simulink model "MIL4L3_SW6_V1_20220211"  (R2018b)
settings: Solver=FixedStepAuto  StartTime=0.0  StopTime=inf  FixedStep=0.001  RelTol=1e-3
PreLoadFcn:
  | A0_MILtest;
undefined symbols (not defined in the file or in its folder): Clb_ICADirect_LaneDisp_StateFive, Clb_ICADirect_LaneDisp_StateFour, Clb_ICADirect_LaneDisp_StateOne, Clb_ICADirect_LaneDisp_StateThree, Clb_ICADirect_LaneDisp_StateTwo, Clb_ICADirect_LaneDisp_StateZero, Clb_ICADirect_LaneDispSW, Clb_ICADirect_TrnLghtsCom_Switch, Clb_ICADirect_TrnLghtsCom_Value, Clb_ICADirect_TrnLghtsCrtl_Inhb, IMAP_Clb_ACU_Driver_Belt, IMAP_Clb_ACU_Driver_Belt_Over, IMAP_Clb_ACU_Passenger_Belt, IMAP_Clb_ACU_Passenger_Belt_Over, IMAP_Clb_ACU_RearLeft_Belt, IMAP_Clb_ACU_RearLeft_Belt_Over, IMAP_Clb_ACU_RearMiddle_Belt, IMAP_Clb_ACU_RearMiddle_Belt_Over, IMAP_Clb_ACU_RearRight_Belt, IMAP_Clb_ACU_RearRight_Belt_Over, IMAP_Clb_AEB_Switch, IMAP_Clb_AEB_Switch_Over, IMAP_Clb_ALC_TLC_Mode, IMAP_Clb_ALC_TLC_Mode_Over, IMAP_Clb_BCM_Battery_Voltage, IMAP_Clb_BCM_Battery_Voltage_Over, IMAP_Clb_BCM_BrakeLamp_State, IMAP_Clb_BCM_BrakeLamp_State_Over, IMAP_Clb_BCM_CHMSL_Status, IMAP_Clb_BCM_CHMSL_Status_Over, IMAP_Clb_BCM_Door_Lock_State, IMAP_Clb_BCM_Door_Lock_State_Over, IMAP_Clb_BCM_FrontWiper_State, IMAP_Clb_BCM_FrontWiper_State_Over, IMAP_Clb_BCM_FrontWiper_Switch, IMAP_Clb_BCM_FrontWiper_Switch_Over, IMAP_Clb_BCM_HazardLamp, IMAP_Clb_BCM_HazardLamp_Over, IMAP_Clb_BCM_HazardLamp_Switch, IMAP_Clb_BCM_HazardLamp_Switch_Over, IMAP_Clb_BCM_HighBeam_State, IMAP_Clb_BCM_HighBeam_State_Over, IMAP_Clb_BCM_Ignition_State, IMAP_Clb_BCM_Ignition_State_Over, IMAP_Clb_BCM_IHBC_Enabled, IMAP_Clb_BCM_IHBC_Enabled_Over, IMAP_Clb_BCM_Left_Light, IMAP_Clb_BCM_Left_Light_Over, IMAP_Clb_BCM_LeftTurn_Switch, IMAP_Clb_BCM_LeftTurn_Switch_Over, IMAP_Clb_BCM_LF_Door_State, IMAP_Clb_BCM_LF_Door_State_Over, IMAP_Clb_BCM_LowBeam_State, IMAP_Clb_BCM_LowBeam_State_Over, IMAP_Clb_BCM_LR_Door_State, IMAP_Clb_BCM_LR_Door_State_Over, IMAP_Clb_BCM_RF_Door_State, IMAP_Clb_BCM_RF_Door_State_Over, IMAP_Clb_BCM_Right_Light, IMAP_Clb_BCM_Right_Light_Over ... (+547)
libraries: CarMaker4SL x2153, simulink x292, dspstat3 x3, canmsglib x2, simulink_extras x1
(part 48 of 52)

== system MIL4L3_SW6_V1_20220211/CarMaker/VehicleControl/Function/LKA/LKAS1/LL/LLOn/LL State Determination (LLStateDet)/LL State Machine Conditions (LLSMCon)/Enable Condition (EnaC)/LKA Own Condition (LKAOwnC)/Vehicle Position Check (VehPosChk)1 ==
  VehPosChk_LaneWidth : Inport
  VehPosChk_bsDvtInfo : Inport  Port=2
  VehPosChk_LKALineMax : Inport  Port=3
  VehPosChk_CarWidth : Inport  Port=4
  VehPosChk_lWarnLineMax_C : Inport  Port=5
  VehPosChk_lWarnLineMin_C : Inport  Port=6
  Bus Selector : BusSelector  OutputSignals=ILftDvt,IRgtDvt
  Logical Operator : Logic  AllPortsSameDT=off  OutDataTypeStr=boolean
  Logical Operator1 : Logic  Operator=OR  AllPortsSameDT=off  OutDataTypeStr=boolean
  Relational Operator1 : RelationalOperator  OutDataTypeStr=boolean  RndMeth=Nearest
  Relational Operator2 : RelationalOperator  OutDataTypeStr=boolean  RndMeth=Nearest
  Relational Operator3 : RelationalOperator  Operator=<=  OutDataTypeStr=boolean  RndMeth=Nearest
  Relational Operator4 : RelationalOperator  Operator=<=  OutDataTypeStr=boolean  RndMeth=Nearest
  Subsystem : Subsystem
  VehPosChk_stVehPosChk : Outport
  VehPosChk_stVehExLane : Outport  Port=2
  wires:
  Bus Selector/1 -> Relational Operator4/1, Relational Operator1/1  "<ILftDvt>"
  Bus Selector/2 -> Relational Operator2/1, Relational Operator3/1  "<IRgtDvt>"
  Relational Operator1/1 -> Logical Operator/1
  Relational Operator2/1 -> Logical Operator/2
  Logical Operator/1 -> VehPosChk_stVehPosChk/1
  VehPosChk_bsDvtInfo/1 -> Bus Selector/1
  Subsystem/1(EnableLine) -> Relational Operator1/2, Relational Operator2/2
  VehPosChk_lWarnLineMax_C/1 -> Subsystem/1(WarnLine_C)
  VehPosChk_LaneWidth/1 -> Subsystem/2(LaneWidth)
  Logical Operator1/1 -> VehPosChk_stVehExLane/1
  Relational Operator3/1 -> Logical Operator1/2
  VehPosChk_lWarnLineMin_C/1 -> Relational Operator3/2, Relational Operator4/2
  Relational Operator4/1 -> Logical Operator1/1
  VehPosChk_LKALineMax/1 -> Subsystem/3(VehPosChk_LKALineMax)
  VehPosChk_CarWidth/1 -> Subsystem/4(VehPosChk_CarWidth)

== system MIL4L3_SW6_V1_20220211/CarMaker/VehicleControl/Function/LKA/LKAS1/LL/LLOn/LL State Determination (LLStateDet)/LL State Machine Conditions (LLSMCon)/Enable Condition (EnaC)/Lane Condition (LaneC)/Lane C1 Detection (LaneC1Det) ==
  LaneWDet_facmL0C1 : Inport
  LaneWDet_facmR0C1 : Inport  Port=2
  Abs : Abs
  Add : Sum  Inputs=+-  OutDataTypeStr=single
  Compare To Constant1 : simulink/Logic and Bit Operations/Compare To Constant  relop=<=  const=0.025  OutDataTypeStr=boolean
  LaneC1Det_stLaneC1DetFlg : Outport
  wires:
  LaneWDet_facmR0C1/1 -> Add/2
  LaneWDet_facmL0C1/1 -> Add/1
  Add/1 -> Abs/1
  Compare To Constant1/1 -> LaneC1Det_stLaneC1DetFlg/1
  Abs/1 -> Compare To Constant1/1

== system MIL4L3_SW6_V1_20220211/CarMaker/VehicleControl/Function/LKA/LKAS1/LL/LLOn/LL State Determination (LLStateDet)/LL State Machine Conditions (LLSMCon)/Enable Condition (EnaC)/Lane Condition (LaneC)/Lane Condition Synthesis (LaneCSyn) ==
  LaneCSyn_stLaneQlECFlg : Inport
  LaneCSyn_stLaneWDetFlg : Inport  Port=2
  LaneCSyn_stLaneCrvtDetFlg : Inport  Port=3
  LaneCSyn_stLaneC1DetFlg : Inport  Port=4
  Logical Operator3 : Logic  Inputs=4  AllPortsSameDT=off  OutDataTypeStr=boolean
  LaneCSyn_stLaneCSyn : Outport
  wires:
  LaneCSyn_stLaneQlECFlg/1 -> Logical Operator3/1
  LaneCSyn_stLaneCrvtDetFlg/1 -> Logical Operator3/3
  Logical Operator3/1 -> LaneCSyn_stLaneCSyn/1
  LaneCSyn_stLaneWDetFlg/1 -> Logical Operator3/2
  LaneCSyn_stLaneC1DetFlg/1 -> Logical Operator3/4

== system MIL4L3_SW6_V1_20220211/CarMaker/VehicleControl/Function/LKA/LKAS1/LL/LLOn/LL State Determination (LLStateDet)/LL State Machine Conditions (LLSMCon)/Enable Condition (EnaC)/Lane Condition (LaneC)/Lane Curvature Detection (LaneCrvtDet) ==
  LaneCrvtDet_crPrvwCrvt : Inport
  LaneCrvtDet_crLaneCrvtMax_C : Inport  Port=2
  Abs : Abs
  Constant : Constant  Value=0  OutDataTypeStr=single  SampleTime=-1
  Interval Test Dynamic : simulink/Logic and Bit Operations/Interval Test Dynamic  IntervalClosedRight=on  IntervalClosedLeft=on  OutDataTypeStr=boolean
      settings: SourceProductName=Simulink  SourceProductBaseCode=SL
  LaneCrvtDet_stLaneCrvtDetFlg : Outport
  wires:
  Interval Test Dynamic/1 -> LaneCrvtDet_stLaneCrvtDetFlg/1
  LaneCrvtDet_crLaneCrvtMax_C/1 -> Interval Test Dynamic/1
  Constant/1 -> Interval Test Dynamic/3
  LaneCrvtDet_crPrvwCrvt/1 -> Abs/1
  Abs/1 -> Interval Test Dynamic/2

== system MIL4L3_SW6_V1_20220211/CarMaker/VehicleControl/Function/LKA/LKAS1/LL/LLOn/LL State Determination (LLStateDet)/LL State Machine Conditions (LLSMCon)/Enable Condition (EnaC)/Lane Condition (LaneC)/Lane Quality Enable Condition (LaneQlEC) ==
  LaneQlEC_stFacmL0Ql : Inport
  LaneQlEC_stFacmR0Ql : Inport  Port=2
  Compare To Constant : simulink/Logic and Bit Operations/Compare To Constant  relop=>  const=2  OutDataTypeStr=boolean
  Compare To Constant1 : simulink/Logic and Bit Operations/Compare To Constant  relop=>  const=2  OutDataTypeStr=boolean
  Logical Operator : Logic  AllPortsSameDT=off  OutDataTypeStr=boolean
  LaneQlEC_stLaneQlECFlg : Outport
  wires:
  LaneQlEC_stFacmL0Ql/1 -> Compare To Constant/1
  LaneQlEC_stFacmR0Ql/1 -> Compare To Constant1/1
  Compare To Constant/1 -> Logical Operator/1
  Compare To Constant1/1 -> Logical Operator/2
  Logical Operator/1 -> LaneQlEC_stLaneQlECFlg/1

== system MIL4L3_SW6_V1_20220211/CarMaker/VehicleControl/Function/LKA/LKAS1/LL/LLOn/LL State Determination (LLStateDet)/LL State Machine Conditions (LLSMCon)/Enable Condition (EnaC)/Lane Condition (LaneC)/Lane Width Detection (LaneWDet) ==
  LaneWDet_LaneWidth : Inport
  LaneWDet_lLaneWMax : Inport  Port=2
  LaneWDet_lLaneWMin : Inport  Port=3
  Abs1 : Abs
  Interval Test Dynamic : simulink/Logic and Bit Operations/Interval Test Dynamic  IntervalClosedRight=on  IntervalClosedLeft=on  OutDataTypeStr=boolean
      settings: SourceProductName=Simulink  SourceProductBaseCode=SL
  LaneWDet_stLaneWDetFlg : Outport
  wires:
  Interval Test Dynamic/1 -> LaneWDet_stLaneWDetFlg/1
  LaneWDet_lLaneWMax/1 -> Interval Test Dynamic/1
  LaneWDet_lLaneWMin/1 -> Interval Test Dynamic/3
  Abs1/1 -> Interval Test Dynamic/2
  LaneWDet_LaneWidth/1 -> Abs1/1

== system MIL4L3_SW6_V1_20220211/CarMaker/VehicleControl/Function/LKA/LKAS1/LL/LLOn/LL State Determination (LLStateDet)/LL State Machine Conditions (LLSMCon)/Enable Condition (EnaC)/Vehicle State Condition (VehStateC)/Emergency Light Enable Condition (EmgcyLghtEC) ==
  EmgcyLghtEC_bsStLampState : Inport
  Add : Sum
  Bus Selector : BusSelector  OutputSignals=BCM_Double_Light,BCM_Left_Light,BCM_Right_Light
  Compare To Constant : simulink/Logic and Bit Operations/Compare To Constant  relop=<=  const=0  OutDataTypeStr=boolean
  Compare To Constant1 : simulink/Logic and Bit Operations/Compare To Constant  relop=>=  const=3  OutDataTypeStr=boolean
  Compare To Constant2 : simulink/Logic and Bit Operations/Compare To Constant  relop=>  const=0  OutDataTypeStr=boolean
  Compare To Constant3 : simulink/Logic and Bit Operations/Compare To Constant  relop=>  const=0  OutDataTypeStr=boolean
  Constant : Constant  Value=3  OutDataTypeStr=single
  Constant1 : Constant  Value=-1  OutDataTypeStr=single
  Logical Operator : Logic  Operator=OR  Inputs=3  AllPortsSameDT=off  OutDataTypeStr=boolean
  Memory : Memory  InheritSampleTime=on
  Saturation : Saturate  UpperLimit=200  LowerLimit=-1
      settings: AttributesFormatString="Min = %<LowerLimit>  Max = %<UpperLimit>"
  Switch : Switch  Criteria=u2 > Threshold
  EmgcyLghtEC_stEmgcyLghtECFlg : Outport
  wires:
  Compare To Constant2/1 -> Logical Operator/2
  Compare To Constant1/1 -> Logical Operator/1
  EmgcyLghtEC_bsStLampState/1 -> Bus Selector/1
  Bus Selector/1 -> Compare To Constant1/1  "<BCM_Double_Light>"
  Bus Selector/2 -> Compare To Constant2/1  "<BCM_Left_Light>"
  Logical Operator/1 -> Switch/2
  Constant/1 -> Switch/1
  Constant1/1 -> Switch/3
  Switch/1 -> Add/1
  Add/1 -> Saturation/1
  Saturation/1 -> Compare To Constant/1, Memory/1
  Memory/1 -> Add/2
  Compare To Constant/1 -> EmgcyLghtEC_stEmgcyLghtECFlg/1
  Bus Selector/3 -> Compare To Constant3/1  "<BCM_Right_Light>"
  Compare To Constant3/1 -> Logical Operator/3

== system MIL4L3_SW6_V1_20220211/CarMaker/VehicleControl/Function/LKA/LKAS1/LL/LLOn/LL State Determination (LLStateDet)/LL State Machine Conditions (LLSMCon)/Enable Condition (EnaC)/Vehicle State Condition (VehStateC)/Gear Enable Condition (GearEC) ==
  GearEC_bsTCUState : Inport
  Bus Selector : BusSelector  OutputSignals=TCU_ActualGear
  Compare To Constant : simulink/Logic and Bit Operations/Compare To Constant  relop===  const=3  OutDataTypeStr=boolean
  GearEC_stGearECFlg : Outport
  wires:
  GearEC_bsTCUState/1 -> Bus Selector/1
  Bus Selector/1 -> Compare To Constant/1  "<TCU_ActualGear>"
  Compare To Constant/1 -> GearEC_stGearECFlg/1

== system MIL4L3_SW6_V1_20220211/CarMaker/VehicleControl/Function/LKA/LKAS1/LL/LLOn/LL State Determination (LLStateDet)/LL State Machine Conditions (LLSMCon)/Enable Condition (EnaC)/Vehicle State Condition (VehStateC)/Vehicle Speed Enable Condition (VehSpdEC) ==
  VehSpdEC_stDACMode : Inport
  VehSpdEC_vVehSpd : Inport  Port=2
  VehSpdEC_vLDWVehSpdMax_C : Inport  Port=3
  VehSpdEC_vLKAVehSpdMax_C : Inport  Port=4
  VehSpdEC_vVehSpdMin_C : Inport  Port=5
  Interval Test Dynamic : simulink/Logic and Bit Operations/Interval Test Dynamic  IntervalClosedRight=on  IntervalClosedLeft=on  OutDataTypeStr=boolean
      settings: SourceProductName=Simulink  SourceProductBaseCode=SL
  Switch : Switch  Threshold=2
  VehSpdEC_stVehSpdECFlg : Outport
  wires:
  VehSpdEC_vVehSpd/1 -> Interval Test Dynamic/2
  VehSpdEC_vVehSpdMin_C/1 -> Interval Test Dynamic/3
  Interval Test Dynamic/1 -> VehSpdEC_stVehSpdECFlg/1
  VehSpdEC_stDACMode/1 -> Switch/2
  VehSpdEC_vLKAVehSpdMax_C/1 -> Switch/1
  Switch/1 -> Interval Test Dynamic/1
  VehSpdEC_vLDWVehSpdMax_C/1 -> Switch/3

== system MIL4L3_SW6_V1_20220211/CarMaker/VehicleControl/Function/LKA/LKAS1/LL/LLOn/LL State Determination (LLStateDet)/LL State Machine Conditions (LLSMCon)/Enable Condition (EnaC)/Vehicle State Condition (VehStateC)/Vehicle State Condition Synthesis (VehStateCSyn) ==
  VehStateCSyn_stVehSpdECFlg : Inport
  VehStateCSyn_stEmgcyLghtECFlg : Inport  Port=2
  VehStateCSyn_stGearECFlg : Inport  Port=3
  Logical Operator : Logic  Inputs=3  AllPortsSameDT=off  OutDataTypeStr=boolean
  VehStateCSyn_stVehStateCSyn : Outport
  wires:
  VehStateCSyn_stVehSpdECFlg/1 -> Logical Operator/1
  VehStateCSyn_stGearECFlg/1 -> Logical Operator/3
  Logical Operator/1 -> VehStateCSyn_stVehStateCSyn/1
  VehStateCSyn_stEmgcyLghtECFlg/1 -> Logical Operator/2

== system MIL4L3_SW6_V1_20220211/CarMaker/VehicleControl/OMAP/OMAP1/Runnable_OMAP_10ms_sys/OMAP_Module/ICA_Direct_G59/ICA_Define/Subsystem1/Dspl/DsplPrcs/Icon ==
  note: 0：灭
      | 1：灰
      | 2：绿
      | 3：橙
      | 4：红
  note: 显示0条件：多车道模式选择ICA；
      | 显示1条件（灰色）：多车道模式选择TCL或ALC，THState~=0；
      | 显示2条件（绿色，不带AUTO）：多车道模式选择TLC，速度大于变道允许门槛值，THState=3；
      | 显示3条件（绿色，带AUTO）：多车道模式选择ALC，速度大于变道允许门槛值，THState=3；
      | 显示4条件（橙色）：多车道模式选择TLC或者ALC，速度大于变道允许门槛值，THState=4
      | 显示5条件（红色）：多车道模式选择TLC或者ALC，速度大于变道允许门槛值，THState=5
      | 之所以把速度条件加进来，其实是考虑到多车道功能的激活隐含了速度要大于某一门槛值这个条件
  note: 0：Default Value
      | 1：HWA Unavailable（未启用）
      | 2：HWA_TLC（触发式变道）
      | 3：HWA_ALC（主动变道）
      | 4：HWA_SL_SRR_Fail（硬件故障-功能无法开启或降级）
      | 5：HWA_Error（系统故障）
      | 6：Reserved（保留）
  note: 0 ：可以从降级回到正常，
      | 1 ：不可以从降级回到正常
  note: ACC_State【0：初始化；1：关闭；2：禁止；3：等待；4：激活；5：Override；6：只能制动；7：Cancel键退出；8：OFF键退出；15：故障】
  Icon_stTHState : Inport
  Icon_stACCState : Inport  Port=2
  Icon_dDgrdIconWarnHiDurnum : Inport  Port=3
  Icon_dDgrdIconWarnLoDurnum : Inport  Port=4
  Icon_dDgrdIconWarnflag : Inport  Port=5
  Icon_stTLC_ALCmodeSW : Inport  Port=6
  Icon_stLC_SpdCndtFlg : Inport  Port=7
  Bus Creator : BusCreator  Inputs=2
  Constant : Constant  Value=OMAP_ICA_iconSTATE0  OutDataTypeStr=uint16
  Constant1 : Constant  Value=OMAP_ICA_iconSTATE1  OutDataTypeStr=uint16
  Constant10 : Constant  Value=5  OutDataTypeStr=uint16
  Constant11 : Constant  OutDataTypeStr=uint16
  Constant12 : Constant  Value=0  OutDataTypeStr=uint16
  Constant13 : Constant  Value=OMAP_ICA_iconSTATE6  OutDataTypeStr=uint16
  Constant14 : Constant  Value=OMAP_ICA_iconSTATE7  OutDataTypeStr=uint16
  Constant15 : Constant  Value=OMAP_ICA_iconSTATE8  OutDataTypeStr=uint16
  Constant16 : Constant  Value=OMAP_ICA_iconSTATE4  OutDataTypeStr=uint16
  Constant2 : Constant  Value=OMAP_ICA_iconSTATE2  OutDataTypeStr=uint16
  Constant3 : Constant  Value=OMAP_ICA_iconSTATE3  OutDataTypeStr=uint16
  Constant4 : Constant  Value=OMAP_ICA_iconSTATE4  OutDataTypeStr=uint16
  Constant5 : Constant  Value=OMAP_ICA_iconSTATE5  OutDataTypeStr=uint16
  Constant6 : Constant  OutDataTypeStr=boolean
  Constant7 : Constant  Value=2  OutDataTypeStr=uint16
  Constant8 : Constant  Value=3  OutDataTypeStr=uint16
  Constant9 : Constant  Value=4  OutDataTypeStr=uint16
  If : If  NumInputs=2  IfExpression=u1==0  ElseIfExpressions=u1==1,u1==2,u1==3,u1==4,u1==5,u1==6,u1==7,(u1==8)&(u2~=4&u2~=5&u2~=6),(u1==8)&(u2==4|u2==5|u2==6)
  If Action Subsystem : Subsystem  TreatAsAtomicUnit=on
  If Action Subsystem1 : Subsystem  TreatAsAtomicUnit=on
  If Action Subsystem10 : Subsystem  TreatAsAtomicUnit=on
  If Action Subsystem11 : Subsystem  TreatAsAtomicUnit=on
  If Action Subsystem12 : Subsystem  TreatAsAtomicUnit=on
  If Action Subsystem13 : Subsystem  TreatAsAtomicUnit=on
  If Action Subsystem14 : Subsystem  TreatAsAtomicUnit=on
  If Action Subsystem15 : Subsystem  TreatAsAtomicUnit=on
  If Action Subsystem16 : Subsystem  TreatAsAtomicUnit=on
  If Action Subsystem2 : Subsystem  TreatAsAtomicUnit=on
  If Action Subsystem3 : Subsystem  TreatAsAtomicUnit=on
  If Action Subsystem4 : Subsystem  TreatAsAtomicUnit=on
  If Action Subsystem5 : Subsystem  TreatAsAtomicUnit=on
  If Action Subsystem6 : Subsystem  TreatAsAtomicUnit=on
  If Action Subsystem7 : Subsystem  TreatAsAtomicUnit=on
  If Action Subsystem8 : Subsystem  TreatAsAtomicUnit=on
  If Action Subsystem9 : Subsystem  TreatAsAtomicUnit=on
  If1 : If  IfExpression=u1 == 0
  If2 : If  NumInputs=3  IfExpression=u1==3&u2==2&u3==1  ElseIfExpressions=u1==3&u2==3&u3==1,u1==4&(u2==2|u2==3)&u3==1,u1==5&(u2==2|u2==3)&u3==1,u1~=0&(u2==2|u2==3)
  Merge : Merge  Inputs=11
  Merge1 : Merge
  Merge2 : Merge  Inputs=6
  Terminator : Terminator
  Terminator1 : Terminator
  Terminator2 : Terminator
  Unit Delay1 : UnitDelay  SampleTime=-1
  else : Subsystem  TreatAsAtomicUnit=on
  if : Subsystem  TreatAsAtomicUnit=on
  Icon_stIconDspl : Outport
  wires:
  Icon_stTHState/1 -> If2/1, If/1
  Icon_stACCState/1 -> If/2
  If/4 -> If Action Subsystem9/Action
  If/2 -> If Action Subsystem7/Action
  If/1 -> If Action Subsystem6/Action
  If/11 -> If Action Subsystem15/Action
  If/3 -> If Action Subsystem8/Action
  If/5 -> If Action Subsystem10/Action
  If Action Subsystem9/1(Out1) -> Merge/4
  Merge/1 -> Bus Creator/1, Unit Delay1/1  "Icon_stICAIcon"
  Unit Delay1/1 -> If Action Subsystem12/1(In1), If Action Subsystem15/1(In1), If Action Subsystem13/1(In1)
  If Action Subsystem6/1(Out1) -> Merge/1
  If Action Subsystem7/1(Out1) -> Merge/2
  If Action Subsystem8/1(Out1) -> Merge/3
  If Action Subsystem10/1(Out1) -> Merge/5
  If Action Subsystem11/1(Out1) -> Merge/6
  Constant/1 -> If Action Subsystem6/1(In1)
  Constant4/1 -> If Action Subsystem10/1(In1)
  Constant1/1 -> If Action Subsystem7/1(In1)
  Constant2/1 -> If Action Subsystem8/1(In1)
  If1/1 -> if/Action
  If1/2 -> else/Action
  Constant6/1 -> if/1(In1)
  if/1(Out1) -> Merge1/1
  Merge1/1 -> Terminator/1  "orange_enable"
  else/2(counter_status) -> Merge1/2
  Icon_dDgrdIconWarnflag/1 -> If1/1  "DgrdIconWarnflag"
  Icon_dDgrdIconWarnHiDurnum/1 -> else/1(HiDurnum)  "DgrdIconWarnHinum"
  Icon_dDgrdIconWarnLoDurnum/1 -> else/2(LoDurnum)  "DgrdIconWarnLonum"
  Icon_stTLC_ALCmodeSW/1 -> If2/2  "DgrdIconWarnLonum"
  Icon_stLC_SpdCndtFlg/1 -> If2/3  "DgrdIconWarnLonum"
  If2/1 -> If Action Subsystem/Action
  Constant7/1 -> If Action Subsystem/1(In1)
  If Action Subsystem/1(Out1) -> Merge2/1
  Constant8/1 -> If Action Subsystem1/1(In1)
  If2/2 -> If Action Subsystem1/Action
  If Action Subsystem1/1(Out1) -> Merge2/2
  Constant9/1 -> If Action Subsystem2/1(In1)
  If2/3 -> If Action Subsystem2/Action
  If Action Subsystem2/1(Out1) -> Merge2/3
  Constant10/1 -> If Action Subsystem3/1(In1)
  If2/4 -> If Action Subsystem3/Action
  If Action Subsystem3/1(Out1) -> Merge2/4
  Constant11/1 -> If Action Subsystem4/1(In1)
  If2/5 -> If Action Subsystem4/Action
  If Action Subsystem4/1(Out1) -> Merge2/5
  Constant12/1 -> If Action Subsystem5/1(In1)
  If2/6 -> If Action Subsystem5/Action
  If Action Subsystem5/1(Out1) -> Merge2/6
  Merge2/1 -> Bus Creator/2  "Icon_stHWAmode"
  Bus Creator/1 -> Icon_stIconDspl/1
  Constant3/1 -> If Action Subsystem9/1(In1)
  Constant5/1 -> If Action Subsystem11/1(In1)
  If/6 -> If Action Subsystem11/Action
  If/7 -> If Action Subsystem12/Action
  If Action Subsystem12/1(Out1) -> Merge/7
  If/8 -> If Action Subsystem13/Action
  If Action Subsystem13/1(Out1) -> Merge/8
  Constant15/1 -> If Action Subsystem14/1(In1)
  If/9 -> If Action Subsystem14/Action
  If Action Subsystem14/1(Out1) -> Merge/9
  If Action Subsystem15/1(Out1) -> Merge/11
  Constant13/1 -> Terminator1/1
  Constant14/1 -> Terminator2/1
  Constant16/1 -> If Action Subsystem16/1(In1)
  If/10 -> If Action Subsystem16/Action
  If Action Subsystem16/1(Out1) -> Merge/10

== system MIL4L3_SW6_V1_20220211/CarMaker/VehicleControl/OMAP/OMAP1/Runnable_OMAP_10ms_sys/OMAP_Module/ICA_Direct_G59/ICA_Define/Subsystem1/Dspl/DsplPrcs/Lane ==
  note: 变道但条件不满足的车道线显示：
      | 1、多车道模式为TLC或者ALC；
      | 1、转向灯已经打了；
      | 2、由于条件不满足，THmode无法跳到状态4（=1或2）；
      | 3、驾驶员没有自己打方向变道（通过接管信号判断），此条其实可以由THState=3覆盖
      | 4、THState在状态3
  note: ->1
  note: ->14
  note: ->2
  note: ->0
  note: 0是运动，1是静止
  Lane_stTHState : Inport
  Lane_stVehSty : Inport  Port=2
  Lane_facmL0Ql : Inport  Port=3
  Lane_facmR0Ql : Inport  Port=4
  Lane_facmL0Type : Inport  Port=5
  Lane_facmR0Type : Inport  Port=6
  Lane_stturn_lightState : Inport  Port=7
  Lane_stTLC_ALCmodeSW : Inport  Port=8
  Lane_stTkOvStChk : Inport  Port=9
  Bus Creator : BusCreator  Inputs=3
  Compare To Constant : simulink/Logic and Bit Operations/Compare To Constant  relop===  const=2  OutDataTypeStr=boolean
  Compare To Constant1 : simulink/Logic and Bit Operations/Compare To Constant  relop===  const=3  OutDataTypeStr=boolean
  Compare To Constant2 : simulink/Logic and Bit Operations/Compare To Constant  relop===  const=3  OutDataTypeStr=boolean
  Compare To Constant3 : simulink/Logic and Bit Operations/Compare To Constant  relop===  const=uint16(3)  OutDataTypeStr=boolean
  Compare To Constant4 : simulink/Logic and Bit Operations/Compare To Constant  relop===  const=uint16(3)  OutDataTypeStr=boolean
  Compare To Constant5 : simulink/Logic and Bit Operations/Compare To Constant  relop===  const=0  OutDataTypeStr=boolean
  Compare To Constant6 : simulink/Logic and Bit Operations/Compare To Constant  relop=~=  const=0  OutDataTypeStr=boolean
  Compare To Zero : simulink/Logic and Bit Operations/Compare To Zero  relop===  OutDataTypeStr=boolean
  Constant{,1,5,13} (4 alike) : Constant  Value=Clb_ICADirect_LaneDisp_StateZero  OutDataTypeStr=uint16
  Constant10 : Constant  OutDataTypeStr=uint16
  Constant11 : Constant  Value=16  OutDataTypeStr=uint16
  Constant12 : Constant  Value=0  OutDataTypeStr=uint16
  Constant14 : Constant  Value=Clb_ICADirect_LaneDisp_StateTwo  OutDataTypeStr=uint16
  Constant15 : Constant  Value=Clb_ICADirect_LaneDisp_StateFive  OutDataTypeStr=uint16
  Constant16 : Constant  Value=Clb_ICADirect_LaneDisp_StateThree  OutDataTypeStr=uint16
  Constant17 : Constant  Value=Clb_ICADirect_LaneDisp_StateFour  OutDataTypeStr=uint16
  Constant18 : Constant  Value=Clb_ICADirect_LaneDispSW  OutDataTypeStr=boolean
  Constant2 : Constant  Value=Clb_ICADirect_LaneDisp_StateTwo  OutDataTypeStr=uint16
  Constant3 : Constant  Value=15  OutDataTypeStr=uint16
  Constant4 : Constant  Value=Clb_ICADirect_LaneDisp_StateOne  OutDataTypeStr=uint16
  Constant6 : Constant  Value=Clb_ICADirect_LaneDisp_StateOne  OutDataTypeStr=uint16
  Constant7 : Constant  Value=3  OutDataTypeStr=uint16
  Constant8 : Constant  OutDataTypeStr=uint16
  Constant9 : Constant  Value=3  OutDataTypeStr=uint16
  Data Type Conversion{,1..7} (8 alike) : DataTypeConversion  OutDataTypeStr=uint16
  If : If  IfExpression=u1==0|u1==5  ElseIfExpressions=u1==3,(u1==1|u1==2|u1==4|u1==6|u1==7|u1==8)
  If1 : If  NumInputs=3  IfExpression=u1==0|u1==5  ElseIfExpressions=u1==3,u1==1|u1==4|(u2<3&u3<3),u2==3&u3==3,u2==3&u3<3,u2<3&u3==3
  Index Vector : MultiPortSwitch  DataPortOrder=Zero-based contiguous  Inputs=2  zeroidx=on
  Logical Operator : Logic  Operator=OR  AllPortsSameDT=off  OutDataTypeStr=boolean
  Logical Operator1 : Logic  Inputs=4  AllPortsSameDT=off  OutDataTypeStr=boolean
  Merge : Merge  Inputs=4
  Merge1 : Merge  Inputs=4
  Merge2 : Merge  Inputs=4
  Merge3 : Merge  Inputs=7
  Multiport Switch : MultiPortSwitch  Inputs=2  DataPortIndices={1,2}  DataPortForDefault=Additional data port  DiagnosticForDefault=None
  Subsystem : Subsystem
  Switch : Switch  Criteria=u2 ~= 0
  Switch1 : Switch  Criteria=u2 ~= 0
  Switch2 : Switch  Criteria=u2 ~= 0
  Switch3 : Switch  Criteria=u2 > Threshold  OutDataTypeStr=uint16
  both_blue : Subsystem  TreatAsAtomicUnit=on
  both_gray1 : Subsystem  TreatAsAtomicUnit=on
  not_dispay : Subsystem  TreatAsAtomicUnit=on
  not_dispay1 : Subsystem  TreatAsAtomicUnit=on
  not_dispay2 : Subsystem  TreatAsAtomicUnit=on
  not_dispay3 : Subsystem  TreatAsAtomicUnit=on
  not_dispay4 : Subsystem  TreatAsAtomicUnit=on
  not_dispay5 : Subsystem  TreatAsAtomicUnit=on
  not_dispay6 : Subsystem  TreatAsAtomicUnit=on
  not_dispay7 : Subsystem  TreatAsAtomicUnit=on
  not_display2 : Subsystem  TreatAsAtomicUnit=on
  Lane_stLaneDspl : Outport
  wires:
  If/1 -> not_dispay/Action
  Lane_stVehSty/1 -> Data Type Conversion1/1
  both_gray1/1(Out1) -> Merge/3
  Lane_facmR0Type/1 -> Compare To Constant4/1
  Lane_facmR0Ql/1 -> If1/3
  Switch/1 -> Lane_stLaneDspl/1
  Compare To Zero/1 -> Switch/2, Subsystem/Enable
  Compare To Constant3/1 -> Switch1/2
  not_display2/1(Out1) -> Merge/4
  Lane_facmL0Type/1 -> Compare To Constant3/1
  Lane_facmL0Ql/1 -> If1/2
  Data Type Conversion5/1 -> Bus Creator/3  "stR0DispType"
  not_dispay/1(Out1) -> Merge/1
  [stL0DispType] -> both_blue/2(In2)
  Compare To Constant4/1 -> Switch2/2
  Constant2/1 -> both_blue/1(In1)
  both_blue/1(Out1) -> Merge/2
  Switch1/1 -> [stL0DispType]
  Subsystem/1(Out1) -> Switch/3
  [stR0DispType] -> both_blue/3(In3)
  Data Type Conversion4/1 -> Bus Creator/2  "stL0DispType"
  Constant8/1 -> Switch1/3
  Merge2/1 -> Data Type Conversion5/1
  Switch2/1 -> [stR0DispType]
  both_blue/3(Out3) -> Merge2/2
  Lane_stTHState/1 -> Data Type Conversion3/1
  Constant9/1 -> Switch2/1
  Merge1/1 -> Data Type Conversion4/1
  not_display2/3(Out3) -> Merge2/4
  Constant10/1 -> Switch2/3
  If/3 -> both_gray1/Action
  not_dispay/3(Out3) -> Merge2/1
  Constant7/1 -> Switch1/1
  If/2 -> both_blue/Action
  [stL0DispType] -> both_gray1/2(In2)
  If/4 -> not_display2/Action
  not_display2/2(Out2) -> Merge1/4
  Constant/1 -> not_dispay/1(In1)
  Bus Creator/1 -> Switch/1, Subsystem/1(In1)
  both_gray1/2(Out2) -> Merge1/3
  [stR0DispType] -> both_gray1/3(In3)
  Merge/1 -> Index Vector/2  "stLaneDspl"
  Data Type Conversion1/1 -> Compare To Zero/1
  [stR0DispType] -> not_dispay/3(In3)
  not_dispay/2(Out2) -> Merge1/1
  [stL0DispType] -> not_dispay/2(In2)
  [stL0DispType] -> not_display2/2(In2)
  Constant5/1 -> not_display2/1(In1)
  Constant4/1 -> both_gray1/1(In1)
  both_gray1/3(Out3) -> Merge2/3
  both_blue/2(Out2) -> Merge1/2
  [stR0DispType] -> not_display2/3(In3)
  Data Type Conversion/1 -> Bus Creator/1  "stLaneDspl"
  Switch3/1 -> Data Type Conversion/1
  Data Type Conversion2/1 -> Compare To Constant1/1, Compare To Constant/1
  Compare To Constant/1 -> Logical Operator/1
  Compare To Constant1/1 -> Logical Operator/2
  Lane_stTLC_ALCmodeSW/1 -> Data Type Conversion2/1
  Lane_stturn_lightState/1 -> Data Type Conversion6/1
  Lane_stTkOvStChk/1 -> Data Type Conversion7/1
  Data Type Conversion7/1 -> Compare To Constant5/1
  Constant3/1 -> Multiport Switch/2
  Constant11/1 -> Multiport Switch/3
  Constant12/1 -> Multiport Switch/4
  Data Type Conversion6/1 -> Multiport Switch/1
  Logical Operator/1 -> Logical Operator1/1
  Compare To Constant5/1 -> Logical Operator1/2
  Compare To Constant2/1 -> Logical Operator1/3
  Multiport Switch/1 -> Compare To Constant6/1, Switch3/1
  Compare To Constant6/1 -> Logical Operator1/4
  Logical Operator1/1 -> Switch3/2
  If1/1 -> not_dispay1/Action
  Constant1/1 -> not_dispay1/1(In1)
  Data Type Conversion3/1 -> If1/1, Compare To Constant2/1, If/1
  If1/2 -> not_dispay2/Action
  Constant14/1 -> not_dispay2/1(In1)
  If1/3 -> not_dispay3/Action
  Constant6/1 -> not_dispay3/1(In1)
  If1/4 -> not_dispay4/Action
  Constant15/1 -> not_dispay4/1(In1)
  If1/5 -> not_dispay5/Action
  Constant16/1 -> not_dispay5/1(In1)
  If1/6 -> not_dispay6/Action
  Constant17/1 -> not_dispay6/1(In1)
  If1/7 -> not_dispay7/Action
  Constant13/1 -> not_dispay7/1(In1)
  not_dispay1/1(Out1) -> Merge3/1
  not_dispay2/1(Out1) -> Merge3/2
  not_dispay3/1(Out1) -> Merge3/3
  not_dispay4/1(Out1) -> Merge3/4
  not_dispay5/1(Out1) -> Merge3/5
  not_dispay6/1(Out1) -> Merge3/6
  not_dispay7/1(Out1) -> Merge3/7
  Constant18/1 -> Index Vector/1
  Merge3/1 -> Index Vector/3  "stLaneDspl"
  Index Vector/1 -> Switch3/3

== system MIL4L3_SW6_V1_20220211/CarMaker/VehicleControl/OMAP/OMAP1/Runnable_OMAP_10ms_sys/OMAP_Module/ICA_Direct_G59/ICA_Define/Subsystem1/Dspl/DsplPrcs/Txt ==
  note: 0是脱手，1是不脱手
  note: 脱手文字提醒时间门限值，15s
  note: 0是运动，1是静止
  Txt_stStWhlHld : Inport
  Txt_stVehSty : Inport  Port=2
  Txt_bsFromFMCMsg : Inport  Port=3
  Txt_stTHFKeyState : Inport  Port=4
  Txt_dHndOffTxtWarnnum : Inport  Port=5
  Txt_stTHState : Inport  Port=6
  Txt_dTxtLimnum : Inport  Port=7
  Txt_stSWALimFlg : Inport  Port=8
  Txt_tiSWALimFlgDetnum : Inport  Port=9
  Txt_stTkOvStChk : Inport  Port=10
  Txt_tfAddVocCmd : Inport  Port=11
  Bus Creator1 : BusCreator  Inputs=21
  Bus Selector1 : BusSelector  OutputSignals=ACC_State,ACC_HMI_Txt_Disp
  Compare To Constant : simulink/Logic and Bit Operations/Compare To Constant  relop===  const=uint16(3)  OutDataTypeStr=boolean
  Compare To Zero : simulink/Logic and Bit Operations/Compare To Zero  relop===  OutDataTypeStr=boolean
  Compare To Zero1 : simulink/Logic and Bit Operations/Compare To Zero  relop=~=  OutDataTypeStr=boolean
  Compare To Zero2 : simulink/Logic and Bit Operations/Compare To Zero  relop===  OutDataTypeStr=boolean
  Data Type Conversion1 : DataTypeConversion  OutDataTypeStr=uint16
  Data Type Conversion14 : DataTypeConversion  OutDataTypeStr=uint16
  Data Type Conversion2 : DataTypeConversion  OutDataTypeStr=uint16
  HndOffTxtTlimit : Subsystem
  Logical Operator : Logic  AllPortsSameDT=off  OutDataTypeStr=boolean
  Logical Operator1 : Logic  AllPortsSameDT=off  OutDataTypeStr=boolean
  PrioPrcs : MATLAB Function  TreatAsAtomicUnit=on
  Terminator{,1..7} (8 alike) : Terminator
  TxtActv : Subsystem
  TxtCncl : Subsystem
  TxtDegraded : Subsystem
  TxtFromACC : Subsystem
  TxtInactv : Subsystem
  TxtOff : Subsystem
  TxtOffToFault : Subsystem
  TxtOn : Subsystem
  TxtOnToFault : Subsystem
  Txt_Tlimit : Subsystem
  Txt_Tlimit1 : Subsystem
  Txt_Tlimit2 : Subsystem
  Txt_Tlimit3 : Subsystem
  Txt_Tlimit4 : Subsystem
  Txt_Tlimit5 : Subsystem
  Txt_Tlimit6 : Subsystem
  Txt_Tlimit7 : Subsystem
  Unit Delay : UnitDelay  SampleTime=-1
  Txt_stTxtDspl : Outport
  Txt_bsMon : Outport  Port=2
  wires:
  Compare To Zero/1 -> Logical Operator/2
  Txt_dHndOffTxtWarnnum/1 -> HndOffTxtTlimit/3(maxlimit)
  Compare To Zero1/1 -> HndOffTxtTlimit/2(reset)
  HndOffTxtTlimit/1(counter_out) -> Terminator/1
  Txt_stStWhlHld/1 -> Compare To Zero1/1, Compare To Zero/1
  HndOffTxtTlimit/2(counter_status) -> Data Type Conversion14/1
  [HndOffFlg] -> PrioPrcs/1(HndOffFlg)
  Txt_stTHState/1 -> Unit Delay/1, [THState]
  Unit Delay/1 -> [LstTHState]
  [THState] -> PrioPrcs/3(THState)
  [OffFlg] -> PrioPrcs/4(OffFlg)
  PrioPrcs/1(PrioPrcs_TxtDspl) -> Txt_stTxtDspl/1, Bus Creator1/1  "TxtDspl"
  [GoReqFlg] -> PrioPrcs/2(GoReqFlg)
  [TkOvFlg] -> PrioPrcs/5(TkOvFlg)
  [ImmdTkOvFlg] -> PrioPrcs/6(ImmdTkOvFlg)
  [RdrBlkFlg] -> PrioPrcs/7(RdrBlkFlg)
  [OnToFaultFlg] -> PrioPrcs/8(OnToFaultFlg)
  [OffToFaultFlg] -> PrioPrcs/9(OffToFaultFlg)
  [CnclFlg] -> PrioPrcs/10(CnclFlg)
  [OnFlg] -> PrioPrcs/11(OnFlg)
  [ActvFlg] -> PrioPrcs/12(ActvFlg)
  [InactvFlg] -> PrioPrcs/13(InactvFlg)
  [THState] -> Bus Creator1/2  "THState"
  [ACCTxtDspl] -> Bus Creator1/3  "ACCTxtDspl"
  [HndOffFlg] -> Bus Creator1/4  "HndOffFlg"
  [GoReqFlg] -> Bus Creator1/5  "GoReqFlg"
  [OffFlg] -> Bus Creator1/6  "OffFlg"
  [TkOvFlg] -> Bus Creator1/7  "TkOvFlg"
  [ImmdTkOvFlg] -> Bus Creator1/8  "ImmdTkOvFlg"
  [RdrBlkFlg] -> Bus Creator1/9  "RdrBlkFlg"
  [OnToFaultFlg] -> Bus Creator1/10  "OnToFaultFlg"
  [OffToFaultFlg] -> Bus Creator1/11  "OffToFaultFlg"
  [CnclFlg] -> Bus Creator1/12  "CnclFlg"
  [OnFlg] -> Bus Creator1/13  "OnFlg"
  [ActvFlg] -> Bus Creator1/14  "ActvFlg"
  [InactvFlg] -> Bus Creator1/15  "InactvFlg"
  Bus Creator1/1 -> Txt_bsMon/1
  Data Type Conversion14/1 -> [HndOffFlg]
  [THState] -> Compare To Constant/1
  Compare To Constant/1 -> Logical Operator1/2
  Logical Operator/1 -> HndOffTxtTlimit/1(incrcondition)
  Txt_bsFromFMCMsg/1 -> Bus Selector1/1
  Data Type Conversion1/1 -> [ACCTxtDspl]
  Bus Selector1/2 -> Data Type Conversion1/1  "<ACC_HMI_Txt_Disp>"
  Data Type Conversion2/1 -> [ACCState]
  Bus Selector1/1 -> Data Type Conversion2/1  "<ACC_State>"
  [THState] -> TxtOffToFault/1(TxtOffToFault_stTHState)
  [LstTHState] -> TxtOffToFault/2(TxtOffToFault_stLstTHState)
  [ACCState] -> TxtOffToFault/3(TxtOffToFault_stACCState)
  [LstTHState] -> TxtOnToFault/2(TxtOnToFault_stLstTHState)
  [THState] -> TxtOnToFault/1(TxtOnToFault_stTHState)
  [THState] -> TxtCncl/1(TxtCncl_stTHState)
  [LstTHState] -> TxtCncl/2(TxtCncl_stLstTHState)
  [LstTHState] -> TxtOn/2(TxtOn_stLstTHState)
  [THState] -> TxtOn/1(TxtOn_stTHState)
  [LstTHState] -> TxtActv/2(TxtActv_stLstTHState)
  [THState] -> TxtActv/1(TxtActv_stTHState)
  [THState] -> TxtInactv/1(TxtInactv_stTHState)
  Txt_stTHFKeyState/1 -> TxtInactv/2(TxtInactv_stTHFKeyState)
  [LstTHState] -> TxtOff/2(TxtOff_stLstTHState)
  [THState] -> TxtOff/1(TxtOff_stTHState)
  [THState] -> TxtFromACC/1(TxtFromACC_stTHState)
  [LstTHState] -> TxtFromACC/2(TxtFromACC_stLstTHState)
  [ACCTxtDspl] -> TxtFromACC/3(TxtFromACC_stACCTxtDspl)
  TxtFromACC/1(TxtFromACC_stGoReq) -> [GoReqFlg]
  TxtFromACC/2(TxtFromACC_stTkOv) -> [TkOvFlg]
  TxtFromACC/3(TxtFromACC_stImmdTkOv) -> [ImmdTkOvFlg]
  TxtFromACC/4(TxtFromACC_stRdrBlk) -> [RdrBlkFlg]
  Txt_dTxtLimnum/1 -> [TxtLimnum]
  [TxtLimnum] -> Txt_Tlimit/2(maxlimit)
  TxtOff/1(TxtOff_stOff) -> Txt_Tlimit/1(incrcondition)
  Txt_Tlimit/1(counter_status) -> [OffFlg]
  Txt_Tlimit1/1(counter_status) -> [OnToFaultFlg]
  TxtOnToFault/1(TxtOnToFault_stOnToFault) -> Txt_Tlimit1/1(incrcondition)
  [TxtLimnum] -> Txt_Tlimit1/2(maxlimit)
  [TxtLimnum] -> Txt_Tlimit2/2(maxlimit)
  TxtOffToFault/1(TxtOffToFault_stOffToFault) -> Txt_Tlimit2/1(incrcondition)
  Txt_Tlimit2/1(counter_status) -> [OffToFaultFlg]
  Txt_Tlimit3/1(counter_status) -> [CnclFlg]
  TxtCncl/1(TxtCncl_stCncl) -> Txt_Tlimit3/1(incrcondition)
  [TxtLimnum] -> Txt_Tlimit3/2(maxlimit)
  [TxtLimnum] -> Txt_Tlimit4/2(maxlimit)
  TxtOn/1(TxtOn_stOn) -> Txt_Tlimit4/1(incrcondition)
  Txt_Tlimit4/1(counter_status) -> [OnFlg]
  Txt_Tlimit5/1(counter_status) -> [ActvFlg]
  TxtActv/1(TxtActv_stActv) -> Txt_Tlimit5/1(incrcondition)
  [TxtLimnum] -> Txt_Tlimit5/2(maxlimit)
  [TxtLimnum] -> Txt_Tlimit6/2(maxlimit)
  TxtInactv/1(TxtInactv_stInactv) -> Txt_Tlimit6/1(incrcondition)
  Txt_Tlimit6/1(counter_status) -> [InactvFlg]
  Txt_Tlimit6/2(counter_reset) -> TxtInactv/3(TxtInactv_stCntRst)
  Txt_Tlimit/2(counter_reset) -> Terminator1/1
  Txt_Tlimit1/2(counter_reset) -> Terminator2/1
  Txt_Tlimit2/2(counter_reset) -> Terminator3/1
  Txt_Tlimit3/2(counter_reset) -> Terminator4/1
  Txt_Tlimit4/2(counter_reset) -> Terminator5/1
  Txt_Tlimit5/2(counter_reset) -> Terminator6/1
  Txt_stSWALimFlg/1 -> TxtFromACC/4(TxtFromACC_stSWALimFlg)
  Txt_tiSWALimFlgDetnum/1 -> TxtFromACC/5(TxtFromACC_tiSWALimFlgDetnum)
  Txt_stTkOvStChk/1 -> TxtFromACC/6(TxtFromACC_stTkOvStChk)
  Compare To Zero2/1 -> Logical Operator1/1
  Logical Operator1/1 -> Logical Operator/1
  [LstTHState] -> TxtDegraded/2(TxtActv_stLstTHState)
  [TxtLimnum] -> Txt_Tlimit7/2(maxlimit)
  Txt_Tlimit7/1(counter_status) -> [DegradedFlg]
  [THState] -> TxtDegraded/1(TxtActv_stTHState)
  TxtDegraded/1(TxtActv_stDegraded) -> Txt_Tlimit7/1(incrcondition)
  Txt_Tlimit7/2(counter_reset) -> Terminator7/1
  [DegradedFlg] -> Bus Creator1/16  "DegradedFlg"
  [DegradedFlg] -> PrioPrcs/14(DegradedFlg)
  TxtFromACC/5(TxtFromACC_stPressSet) -> [PressSetFlg]
  TxtFromACC/9(TxtFromACC_stISAToOff) -> [ISAToOffFlg]
  TxtFromACC/8(TxtFromACC_stISAToOn) -> [ISAToOnFlg]
  TxtFromACC/7(TxtFromACC_stResBrkPedal) -> [ResBrkPedalFlg]
  TxtFromACC/6(TxtFromACC_stResEPB) -> [ResEPBFlg]
  Txt_tfAddVocCmd/1 -> TxtFromACC/7(TxtFromACC_tfAddVocCmd)
  [ResBrkPedalFlg] -> PrioPrcs/17(ResBrkPedalFlg)
  [ISAToOnFlg] -> PrioPrcs/18(ISAToOnFlg)
  [ISAToOffFlg] -> PrioPrcs/19(ISAToOffFlg)
  [PressSetFlg] -> PrioPrcs/15(PressSetFlg)
  [ResEPBFlg] -> PrioPrcs/16(ResEPBFlg)
  [PressSetFlg] -> Bus Creator1/17  "PressSetFlg"
  [ResEPBFlg] -> Bus Creator1/18  "ResEPBFlg"
  [ResBrkPedalFlg] -> Bus Creator1/19  "ResBrkPedalFlg"
  [ISAToOnFlg] -> Bus Creator1/20  "ISAToOnFlg"
  [ISAToOffFlg] -> Bus Creator1/21  "ISAToOffFlg"
  Txt_stVehSty/1 -> TxtFromACC/8(TxtFromACC_stVehSty), Compare To Zero2/1

== system MIL4L3_SW6_V1_20220211/CarMaker/VehicleControl/OMAP/OMAP1/Runnable_OMAP_10ms_sys/OMAP_Module/ICA_Direct_G59/ICA_Define/Subsystem1/Dspl/DsplPrcs/Voc ==
  note: 功能降级声音提示时长
  Voc_stStWhlHld : Inport
  Voc_stTHState : Inport  Port=2
  Voc_dDgrdVocWarnDurnum : Inport  Port=3
  Voc_dHndOffVocWarnnum : Inport  Port=4
  Voc_stVehSty : Inport  Port=5
  Compare To Constant : simulink/Logic and Bit Operations/Compare To Constant  relop===  const=uint16(3)  OutDataTypeStr=boolean
  Compare To Constant1 : simulink/Logic and Bit Operations/Compare To Constant  relop===  const=uint16(4)  OutDataTypeStr=boolean
  Compare To Constant2 : simulink/Logic and Bit Operations/Compare To Constant  relop===  const=uint16(3)  OutDataTypeStr=boolean
  Compare To Constant3 : simulink/Logic and Bit Operations/Compare To Constant  relop===  const=uint16(4)  OutDataTypeStr=boolean
  Compare To Zero1 : simulink/Logic and Bit Operations/Compare To Zero  relop===  OutDataTypeStr=boolean
  Compare To Zero2 : simulink/Logic and Bit Operations/Compare To Zero  relop===  OutDataTypeStr=boolean
  Data Type Conversion{,1..3} (4 alike) : DataTypeConversion  OutDataTypeStr=uint16
  Logical Operator : Logic  AllPortsSameDT=off  OutDataTypeStr=boolean
  Logical Operator1 : Logic  Inputs=3  AllPortsSameDT=off  OutDataTypeStr=boolean
  Logical Operator3 : Logic  Operator=OR  AllPortsSameDT=off  OutDataTypeStr=boolean
  MATLAB_Function : MATLAB Function  TreatAsAtomicUnit=on
  Sum_Condition : Subsystem  TreatAsAtomicUnit=on
  Switch : Switch  Criteria=u2 ~= 0
  Unit Delay : UnitDelay  SampleTime=-1
  Voc_stVocDspl : Outport
  wires:
  Voc_stTHState/1 -> Compare To Constant3/1, Compare To Constant2/1, Unit Delay/1, Compare To Constant1/1
  Unit Delay/1 -> Compare To Constant/1
  Compare To Constant1/1 -> Logical Operator/1
  Compare To Constant/1 -> Logical Operator/2
  Data Type Conversion/1 -> MATLAB_Function/1(Warning_duration)
  Data Type Conversion1/1 -> MATLAB_Function/2(Trigger)
  MATLAB_Function/1(Warning) -> Switch/2, Switch/1
  Voc_stStWhlHld/1 -> Compare To Zero1/1
  Sum_Condition/1(Out) -> Voc_stVocDspl/1
  Data Type Conversion3/1 -> Sum_Condition/Enable, Sum_Condition/1(In)
  Voc_dHndOffVocWarnnum/1 -> Data Type Conversion2/1
  Data Type Conversion2/1 -> Sum_Condition/2(Sum)
  Compare To Zero1/1 -> Logical Operator1/2
  Logical Operator1/1 -> Data Type Conversion3/1
  Voc_dDgrdVocWarnDurnum/1 -> Data Type Conversion/1
  Voc_stVehSty/1 -> Compare To Zero2/1
  Compare To Zero2/1 -> Logical Operator1/3
  Logical Operator/1 -> Data Type Conversion1/1
  Compare To Constant2/1 -> Logical Operator3/1
  Compare To Constant3/1 -> Logical Operator3/2
  Logical Operator3/1 -> Logical Operator1/1

== system MIL4L3_SW6_V1_20220211/CarMaker/VehicleControl/Function/LKA/LKAS1/LL/LLOn/LKA/LKA Motion Planning (LKAMP) /Switching Condition (SwtCon)/Ending Heading Angle Determination (EndHdAgDet)/Lateral Speed Compensation (LSpdComp)/If Action Subsystem ==
  In1 : Inport
  Action Port : ActionPort  InitializeStates=reset  ActionType=then
      settings: AttributesFormatString=states = %<InitializeStates>
  Cast To Single1 : DataTypeConversion  LockScale=on
  Out1 : Outport  InitialOutput=0
      settings: AttributesFormatString=%<OutputWhenDisabled> = %<InitialOutput>
  wires:
  Cast To Single1/1 -> Out1/1
  In1/1 -> Cast To Single1/1

== system MIL4L3_SW6_V1_20220211/CarMaker/VehicleControl/Function/LKA/LKAS1/LL/LLOn/LKA/LKA Motion Planning (LKAMP) /Switching Condition (SwtCon)/Ending Heading Angle Determination (EndHdAgDet)/Lateral Speed Compensation (LSpdComp)/If Action Subsystem2 ==
  Action Port : ActionPort  InitializeStates=reset  ActionType=else
      settings: AttributesFormatString=states = %<InitializeStates>
  Constant : Constant  Value=0  OutDataTypeStr=single
  Out1 : Outport  InitialOutput=0
      settings: AttributesFormatString=%<OutputWhenDisabled> = %<InitialOutput>
  wires:
  Constant/1 -> Out1/1

== system MIL4L3_SW6_V1_20220211/CarMaker/VehicleControl/Function/LKA/LKAS1/LL/LLOn/LKA/LKA Motion Planning (LKAMP) /Switching Condition (SwtCon)/Ending Heading Angle Determination (EndHdAgDet)/Lateral Speed Compensation (LSpdComp)/If Action Subsystem4 ==
  In1 : Inport
  Action Port : ActionPort  InitializeStates=reset  ActionType=elseif
      settings: AttributesFormatString=states = %<InitializeStates>
  Cast To Single1 : DataTypeConversion  LockScale=on
  Out1 : Outport  InitialOutput=0
      settings: AttributesFormatString=%<OutputWhenDisabled> = %<InitialOutput>
  wires:
  Cast To Single1/1 -> Out1/1
  In1/1 -> Cast To Single1/1

== system MIL4L3_SW6_V1_20220211/CarMaker/VehicleControl/Function/LKA/LKAS1/LL/LLOn/LKA/Lane Following (LF)/Trajectory Following Control (TFC)/Feedback Control (FbCtl)/Subsystem/If Action Subsystem ==
  In1 : Inport
  Action Port : ActionPort  ActionType=then
      settings: AttributesFormatString=states = %<InitializeStates>
  Out1 : Outport
      settings: AttributesFormatString=%<OutputWhenDisabled> = %<InitialOutput>
  wires:
  In1/1 -> Out1/1

== system MIL4L3_SW6_V1_20220211/CarMaker/VehicleControl/Function/LKA/LKAS1/LL/LLOn/LKA/Lane Following (LF)/Trajectory Following Control (TFC)/Feedback Control (FbCtl)/Subsystem/If Action Subsystem1 ==
  In1 : Inport
  Action Port : ActionPort  ActionType=elseif
      settings: AttributesFormatString=states = %<InitializeStates>
  Out1 : Outport
      settings: AttributesFormatString=%<OutputWhenDisabled> = %<InitialOutput>
  wires:
  In1/1 -> Out1/1

== system MIL4L3_SW6_V1_20220211/CarMaker/VehicleControl/Function/LKA/LKAS1/LL/LLOn/LKA/Lane Following (LF)/Trajectory Following Control (TFC)/Feedback Control (FbCtl)/Subsystem/If Action Subsystem2 ==
  In1 : Inport
  Action Port : ActionPort  ActionType=else
      settings: AttributesFormatString=states = %<InitializeStates>
  Out1 : Outport
      settings: AttributesFormatString=%<OutputWhenDisabled> = %<InitialOutput>
  wires:
  In1/1 -> Out1/1

== system MIL4L3_SW6_V1_20220211/CarMaker/VehicleControl/Function/LKA/LKAS1/LL/LLOn/LKA/Lane Following (LF)/Trajectory Following Control (TFC)/Feedback Control (FbCtl)/Subsystem/Signal Latching2 ==
  In : Inport
  Add : Sum  OutDataTypeStr=uint16
  Constant : Constant  OutDataTypeStr=uint16  SampleTime=-1
  Constant2 : Constant  Value=LatchTime  OutDataTypeStr=uint16  SampleTime=-1
  If : If  NumInputs=2  IfExpression=u1==u2  ShowElse=off
  Memory : Memory  InheritSampleTime=on
  Saturation1 : Saturate  UpperLimit=10000  LowerLimit=0  OutDataTypeStr=uint16
  "if action " : Subsystem  TreatAsAtomicUnit=on
  Out : Outport
  wires:
  Constant2/1 -> If/2
  In/1 -> "if action "/1(In)
  "if action "/1(Out) -> Out/1
  If/1 -> "if action "/Action
  Constant/1 -> Add/1
  Add/1 -> Saturation1/1
  Memory/1 -> Add/2
  Saturation1/1 -> Memory/1, If/1

== system MIL4L3_SW6_V1_20220211/CarMaker/VehicleControl/Function/LKA/LKAS1/LL/LLOn/LKA/Plan To LaneFollowing (PTLF)/InsideJudge1/If Action Subsystem/If Action Subsystem/Signal Latching ==
  In : Inport
  Add : Sum  OutDataTypeStr=uint16
  Constant : Constant  OutDataTypeStr=uint16  SampleTime=-1
  Constant2 : Constant  Value=LatchTime  OutDataTypeStr=uint16  SampleTime=-1
  If : If  NumInputs=2  IfExpression=u1<=u2  ShowElse=off
  Memory : Memory  InheritSampleTime=on
  Saturation1 : Saturate  UpperLimit=10000  LowerLimit=0  OutDataTypeStr=uint16
  "if action " : Subsystem  TreatAsAtomicUnit=on
  Out : Outport
  wires:
  Saturation1/1 -> If/1, Memory/1
  Memory/1 -> Add/2
  Add/1 -> Saturation1/1
  Constant/1 -> Add/1
  If/1 -> "if action "/Action
  "if action "/1(Out) -> Out/1
  In/1 -> "if action "/1(In)
  Constant2/1 -> If/2

== system MIL4L3_SW6_V1_20220211/CarMaker/VehicleControl/Function/LKA/LKAS1/LL/LLOn/LKA/Plan To LaneFollowing (PTLF)/InsideJudge1/If Action Subsystem/If Action Subsystem/Signal Latching1 ==
  In : Inport
  Add : Sum  OutDataTypeStr=uint16
  Constant : Constant  OutDataTypeStr=uint16  SampleTime=-1
  Constant2 : Constant  Value=LatchTime  OutDataTypeStr=uint16  SampleTime=-1
  If : If  NumInputs=2  IfExpression=u1==u2  ShowElse=off
  Memory : Memory  InheritSampleTime=on
  Saturation1 : Saturate  UpperLimit=10000  LowerLimit=0  OutDataTypeStr=uint16
  "if action " : Subsystem  TreatAsAtomicUnit=on
  Out : Outport
  wires:
  Constant2/1 -> If/2
  In/1 -> "if action "/1(In)
  "if action "/1(Out) -> Out/1
  If/1 -> "if action "/Action
  Constant/1 -> Add/1
  Add/1 -> Saturation1/1
  Memory/1 -> Add/2
  Saturation1/1 -> Memory/1, If/1

== system MIL4L3_SW6_V1_20220211/CarMaker/VehicleControl/Function/LKA/LKAS1/LL/LLOn/LKA/Plan To LaneFollowing (PTLF)/InsideJudge1/If Action Subsystem1/If Action Subsystem/Signal Latching ==
  In : Inport
  Add : Sum  OutDataTypeStr=uint16
  Constant : Constant  OutDataTypeStr=uint16  SampleTime=-1
  Constant2 : Constant  Value=LatchTime  OutDataTypeStr=uint16  SampleTime=-1
  If : If  NumInputs=2  IfExpression=u1<=u2  ShowElse=off
  Memory : Memory  InheritSampleTime=on
  Saturation1 : Saturate  UpperLimit=10000  LowerLimit=0  OutDataTypeStr=uint16
  "if action " : Subsystem  TreatAsAtomicUnit=on
  Out : Outport
  wires:
  Saturation1/1 -> If/1, Memory/1
  Memory/1 -> Add/2
  Add/1 -> Saturation1/1
  Constant/1 -> Add/1
  If/1 -> "if action "/Action
  "if action "/1(Out) -> Out/1
  In/1 -> "if action "/1(In)
  Constant2/1 -> If/2

== system MIL4L3_SW6_V1_20220211/CarMaker/VehicleControl/Function/LKA/LKAS1/LL/LLOn/LKA/Plan To LaneFollowing (PTLF)/InsideJudge1/If Action Subsystem1/If Action Subsystem/Signal Latching1 ==
  In : Inport
  Add : Sum  OutDataTypeStr=uint16
  Constant : Constant  OutDataTypeStr=uint16  SampleTime=-1
  Constant2 : Constant  Value=LatchTime  OutDataTypeStr=uint16  SampleTime=-1
  If : If  NumInputs=2  IfExpression=u1==u2  ShowElse=off
  Memory : Memory  InheritSampleTime=on
  Saturation1 : Saturate  UpperLimit=10000  LowerLimit=0  OutDataTypeStr=uint16
  "if action " : Subsystem  TreatAsAtomicUnit=on
  Out : Outport
  wires:
  Constant2/1 -> If/2
  In/1 -> "if action "/1(In)
  "if action "/1(Out) -> Out/1
  If/1 -> "if action "/Action
  Constant/1 -> Add/1
  Add/1 -> Saturation1/1
  Memory/1 -> Add/2
  Saturation1/1 -> Memory/1, If/1

== system MIL4L3_SW6_V1_20220211/CarMaker/VehicleControl/Function/LKA/LKAS1/LL/LLOn/LL State Determination (LLStateDet)/LL State Machine Conditions (LLSMCon)/Activation Condition (ActvC)/Deviation Threshold Condition (DvtThresCon)/Deviation Threshold Judgement LDW (DvtThresJdg)/Deviation Speed Detection (DvtSpdDet) ==
  DvtSpdDet_vLftDvtSpd : Inport
  DvtSpdDet_vRgtDvtSpd : Inport  Port=2
  DvtSpdDet_vDvtSpdMin_C : Inport  Port=3
  If : If  NumInputs=3  IfExpression=u1>=u3 & u2>=u3  ElseIfExpressions=u1<=-u3 & u2<=-u3
  Memory : Memory  InheritSampleTime=on
  Merge1 : Merge  Inputs=3
  Ph1SWA : Subsystem
  Ph2SWA : Subsystem
  Ph3SWA : Subsystem
  DvtSpdDet_stDvtSpdFlg : Outport
  wires:
  Memory/1 -> Ph3SWA/1(In1)
  Merge1/1 -> DvtSpdDet_stDvtSpdFlg/1, Memory/1
  If/3 -> Ph3SWA/Action
  If/2 -> Ph2SWA/Action
  Ph3SWA/1(Out) -> Merge1/3
  Ph2SWA/1(Out) -> Merge1/2
  Ph1SWA/1(Out) -> Merge1/1
  If/1 -> Ph1SWA/Action
  DvtSpdDet_vDvtSpdMin_C/1 -> If/3
  DvtSpdDet_vRgtDvtSpd/1 -> If/2
  DvtSpdDet_vLftDvtSpd/1 -> If/1

== system MIL4L3_SW6_V1_20220211/CarMaker/VehicleControl/Function/LKA/LKAS1/LL/LLOn/LL State Determination (LLStateDet)/LL State Machine Conditions (LLSMCon)/Activation Condition (ActvC)/Deviation Threshold Condition (DvtThresCon)/Deviation Threshold Judgement LDW (DvtThresJdg)/Deviation Threshold Condition Synthesis (DTCSyn) ==
  DTCSyn_stLftDvtThresActvFlg : Inport
  DTCSyn_stRgtDvtThresActvFlg : Inport  Port=2
  DTCSyn_stDvtSpdFlg : Inport  Port=3
  Cast To Single : DataTypeConversion  OutDataTypeStr=uint8
  Cast To Single1 : DataTypeConversion  OutDataTypeStr=uint8
  Cast To Single2 : DataTypeConversion  LockScale=on
  Constant2 : Constant  Value=0  OutDataTypeStr=uint8
  Gain1 : Gain  Gain=2  OutDataTypeStr=Inherit: Same as input
  Switch2 : Switch  Criteria=u2 > Threshold
  Switch3 : Switch
  DTCSyn_stDvtThresActvFlg : Outport
  wires:
  Cast To Single1/1 -> Gain1/1
  Cast To Single/1 -> Cast To Single2/1
  Gain1/1 -> Switch3/3  "DvtThresActvFlg"
  Cast To Single2/1 -> Switch2/1  "DvtThresActvFlg"
  Constant2/1 -> Switch2/3  "DvtThresActvFlg"
  DTCSyn_stDvtSpdFlg/1 -> Switch2/2, Switch3/2
  Switch3/1 -> DTCSyn_stDvtThresActvFlg/1
  Switch2/1 -> Switch3/1
  DTCSyn_stLftDvtThresActvFlg/1 -> Cast To Single/1
  DTCSyn_stRgtDvtThresActvFlg/1 -> Cast To Single1/1

== system MIL4L3_SW6_V1_20220211/CarMaker/VehicleControl/Function/LKA/LKAS1/LL/LLOn/LL State Determination (LLStateDet)/LL State Machine Conditions (LLSMCon)/Activation Condition (ActvC)/Deviation Threshold Condition (DvtThresCon)/Deviation Threshold Judgement LDW (DvtThresJdg)/Left Side Deviation Threshold Condition (LftDTC) ==
  LftDTC_bsDvtThresInfo : Inport
  LftDTC_lLftDvt : Inport  Port=2
  LftDTC_vLftDvtSpd : Inport  Port=3
  Abs : Abs
  Bus Selector : BusSelector  OutputSignals=LL_ThresDet_lDvtThresLwrLDW,LL_ThresDet_lDvtThresUprLDW,LL_ThresDet_tiTTLCThresLDW
  Divide : Product  Inputs=**
  Relational Operator2 : RelationalOperator  Operator=<=  OutDataTypeStr=boolean  RndMeth=Nearest
  Saturation Dynamic : simulink/Discontinuities/Saturation Dynamic  OutMin=[]  OutMax=[]  OutDataTypeStr=Inherit: Same as second input  OutDataType=fixdt(1, 16)  OutScaling=2^-10  DoSatur=off
  LftDTC_stLftDvtThresActvFlg : Outport
  wires:
  Abs/1 -> Divide/2
  Saturation Dynamic/1 -> Relational Operator2/2
  Divide/1 -> Saturation Dynamic/2
  LftDTC_vLftDvtSpd/1 -> Abs/1
  LftDTC_lLftDvt/1 -> Relational Operator2/1
  Relational Operator2/1 -> LftDTC_stLftDvtThresActvFlg/1
  Bus Selector/2 -> Saturation Dynamic/1  "<LL_ThresDet_lDvtThresUprLDW>"
  Bus Selector/3 -> Divide/1  "<LL_ThresDet_tiTTLCThresLDW>"
  Bus Selector/1 -> Saturation Dynamic/3  "<LL_ThresDet_lDvtThresLwrLDW>"
  LftDTC_bsDvtThresInfo/1 -> Bus Selector/1
